simulink model "model_2"  (R2021a)
settings: Solver=VariableStepAuto  StartTime=0.0  StopTime=48.0  RelTol=1e-3
settings Model: Creator=alamg  LastModifiedBy=alamg

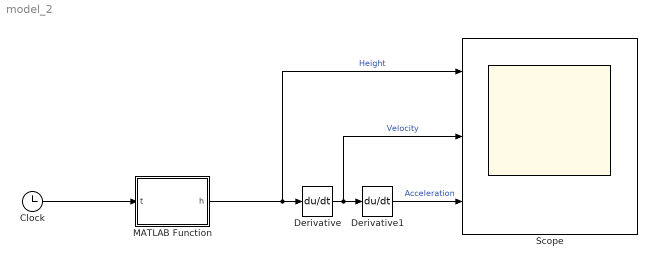
== system model_2 ==
  Clock : Clock
  Derivative : Derivative
  Derivative1 : Derivative
  MATLAB Function : MATLAB Function  TreatAsAtomicUnit=on
  Scope : Scope  NumInputPorts=3
  wires:
  MATLAB Function/1(h) -> Scope/1, Derivative/1  "Height"
  Derivative/1 -> Scope/2, Derivative1/1  "Velocity"
  Derivative1/1 -> Scope/3  "Acceleration"
  Clock/1 -> MATLAB Function/1(t)

== matlab function model_2/MATLAB Function ==
  data: t input; h output
function h = fcn(t)
h = -0.12*t^4 + 12*t^3 - 380*t^2 + 4100*t + 220;
